simulink model "major_project1"  (R2025a)
settings: Solver=VariableStepAuto  StartTime=0.0  StopTime=5  RelTol=1e-3
undefined symbols (not defined in the file): Ion, Lithium
libraries: spsSeriesRLCBranchLib x8, spsMosfetLib x7, spsBatteryLib x3, spsVoltageMeasurementLib x3, spsPVArrayLib x1, slpidlib x1, simulink x1, spspowerguiLib x1
settings Model: Creator=Telan  LastModifiedBy=Telan
settings DataIOCC: SaveFormat=Array
settings DebuggingCC: UnderSpecifiedDimensionMsg=warning

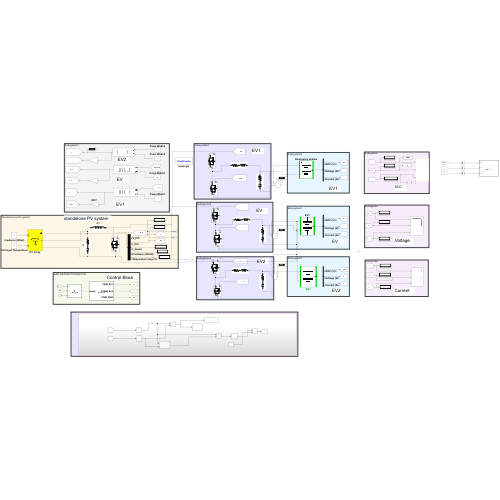
[thumbnail: Simulink's stored preview of the top-level diagram]
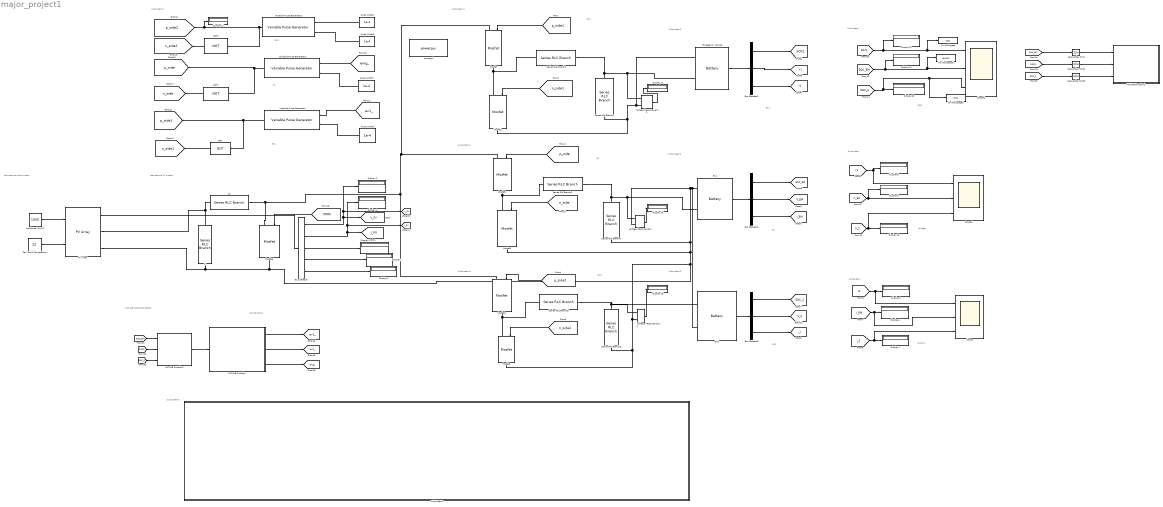
== system major_project1 ==
  note: Subsystem3
  note: EV1
  note: Subsystem
  note: Subsystem
  note: Subsystem
  note: Subsystem1
  note: MATLAB FUNCTION BLOCK
  note: Subsystem5
  note: Subsystem3
  note: Subsystem2
  note: Subsystem4
  note: Standalone solar system
  note: Subsystem4
  note: Subsystem4
  note: EV2
  note: EV
  note: EV1
  note: EV
  note: EV2
  note: SOC
  note: Voltage
  note: Current
  note: EV1
  note: EV
  note: EV2
  note: standalone PV system
  note: Control Block
  Bus Selector : BusSelector  OutputSignals=V_PV,I_PV,I_diode,Irradiance (W/m2),Temperature (deg C)
  Bus Selector1 : BusSelector  OutputSignals=SOC (%),Voltage (V),Current (A)
  Bus Selector2 : BusSelector  OutputSignals=SOC (%),Voltage (V),Current (A)
  Bus Selector3 : BusSelector  OutputSignals=SOC (%),Voltage (V),Current (A)
  C : spsSeriesRLCBranchLib/Series RLC Branch  LConnTagsString=__new0  RConnTagsString=__new0  BranchType=RC  Resistance=0.0001  Inductance=1e-3  SetiL0=off  InitialCurrent=0  Capacitance=988E-6  Setx0=off  InitialVoltage=0  Measurements=Branch voltage and current
  C1 : spsSeriesRLCBranchLib/Series RLC Branch  LConnTagsString=__new0  RConnTagsString=__new0  BranchType=L  Resistance=0.0001  Inductance=1.6e-3  SetiL0=off  InitialCurrent=0  Capacitance=988E-6  Setx0=off  InitialVoltage=0  Measurements=Branch voltage and current
  Cell Input Temperature : Constant  Value=25
  Display{,1..17} (18 alike) : Display
  EV1 : spsBatteryLib/Battery  BatType=Lithium-Ion  NomV=250  NomQ=60  SOC=30  Batt_Tr=5  PresetModel=on  MaxQ=60  MinV=187.5  FullV=290.9968  Dis_rate=26.087  R=0.041667  Normal_OP=54.2609  expZone="[270.0965      2.947826]"
  EV2 : spsBatteryLib/Battery  BatType=Lithium-Ion  NomV=250  NomQ=50  SOC=50  Batt_Tr=5  PresetModel=on  MaxQ=50  MinV=187.5  FullV=290.9968  Dis_rate=21.7391  R=0.05  Normal_OP=45.2174  expZone="[270.0965      2.456522]"
  Emergency Vehicle : spsBatteryLib/Battery  BatType=Lithium-Ion  NomV=250  NomQ=50  SOC=50  Batt_Tr=5  PresetModel=on  MaxQ=50  MinV=187.5  FullV=290.9968  Dis_rate=21.7391  R=0.05  Normal_OP=45.2174  expZone="[270.0965      2.456522]"
  Irradiance (W/m2) : Constant  Value=1000
  MATLAB Function : MATLAB Function  TreatAsAtomicUnit=on
  MATLAB Function1 : MATLAB Function  TreatAsAtomicUnit=on
  MATLAB Function2 : MATLAB Function  TreatAsAtomicUnit=on
  Mosfet{,1..6} (7 alike) : spsMosfetLib/Mosfet  Ron=0.1  Lon=0  Rd=0.01  Vfd=0  IC=0  Rs=1e5  Cs=inf  Measurements=off
  NOT : Logic  Operator=NOT  IconShape=distinctive  AllPortsSameDT=off  OutDataTypeStr=boolean
  NOT1 : Logic  Operator=NOT  IconShape=distinctive  AllPortsSameDT=off  OutDataTypeStr=boolean
  NOT2 : Logic  Operator=NOT  IconShape=distinctive  AllPortsSameDT=off  OutDataTypeStr=boolean
  PV  Array : spsPVArrayLib/PV Array  Npar=40  Nser=10  PlotType=array @ 1000 W/m2 & specified temperatures  S_vec="[ 1000  500  100 ]"  Temp_C_vec="[ 45 25  ]"  ModuleName=User-defined  PlotWhenSelected=off  Pm=213.15  Ncell=60  Voc=36.3  Isc=7.84  Vm=29  Im=7.35  beta_Voc_pc=-0.36099  alpha_Isc_pc=0.102  beta_Voc=-0.13104  alpha_Isc=0.0079968  IL=7.8654  I0=2.9273e-10  nI=0.98119  Rsh=313.0553  Rs=0.39381  RobustModel=off  RobustCellTemperature=313.3991  BAL=on  Tc=1e-6  Tfilter=5e-5
  Pulse Width{1..4} (4 alike) : Constant  Value=1e-4
  Scope : Scope  NumInputPorts=3
      settings: ActiveDisplayYMinimum=-6.4724154503791311  ActiveDisplayYMaximum=55.444981382819826
  Scope1 : Scope  NumInputPorts=3
      settings: ActiveDisplayYMinimum=-33.657064546931281  ActiveDisplayYMaximum=302.91358092238158
  Scope2 : Scope  NumInputPorts=3
      settings: ActiveDisplayYMinimum=51.5865917372177  ActiveDisplayYMaximum=51.68343264048265  DataLoggingVariableName=ScopeData2
  Series RLC Branch1 : spsSeriesRLCBranchLib/Series RLC Branch  LConnTagsString=__new0  RConnTagsString=__new0  BranchType=RL  Resistance=0.1  Inductance=9e-4  SetiL0=off  InitialCurrent=0  Capacitance=1e-6  Setx0=off  InitialVoltage=0  Measurements=None
  Series RLC Branch2 : spsSeriesRLCBranchLib/Series RLC Branch  LConnTagsString=__new0  RConnTagsString=__new0  BranchType=RC  Resistance=30  Inductance=1e-3  SetiL0=off  InitialCurrent=0  Capacitance=1e-4  Setx0=off  InitialVoltage=0  Measurements=Branch voltage
  Series RLC Branch3 : spsSeriesRLCBranchLib/Series RLC Branch  LConnTagsString=__new0  RConnTagsString=__new0  BranchType=RL  Resistance=0.1  Inductance=9e-4  SetiL0=off  InitialCurrent=0  Capacitance=1e-6  Setx0=off  InitialVoltage=0  Measurements=None
  Series RLC Branch4 : spsSeriesRLCBranchLib/Series RLC Branch  LConnTagsString=__new0  RConnTagsString=__new0  BranchType=RC  Resistance=30  Inductance=1e-3  SetiL0=off  InitialCurrent=0  Capacitance=1e-4  Setx0=off  InitialVoltage=0  Measurements=Branch voltage
  Series RLC Branch5 : spsSeriesRLCBranchLib/Series RLC Branch  LConnTagsString=__new0  RConnTagsString=__new0  BranchType=RL  Resistance=0.1  Inductance=9e-4  SetiL0=off  InitialCurrent=0  Capacitance=1e-6  Setx0=off  InitialVoltage=0  Measurements=None
  Series RLC Branch6 : spsSeriesRLCBranchLib/Series RLC Branch  LConnTagsString=__new0  RConnTagsString=__new0  BranchType=RC  Resistance=30  Inductance=1e-3  SetiL0=off  InitialCurrent=0  Capacitance=1e-4  Setx0=off  InitialVoltage=0  Measurements=Branch voltage
  Subsystem2 : Subsystem
  To Workspace : ToWorkspace  VariableName=soc1  SampleTime=1
      settings: Save2DSignal=2-D array (concatenate along first dimension)
  To Workspace1 : ToWorkspace  VariableName=soc_em  SampleTime=-1
      settings: Save2DSignal=2-D array (concatenate along first dimension)
  To Workspace2 : ToWorkspace  VariableName=soc2  SampleTime=-1
      settings: Save2DSignal=2-D array (concatenate along first dimension)
  Variable Pulse Generator : VariablePulseGenerator  AllowZeroPulseWidth=on  SampleTime=0.1
  Variable Pulse Generator1 : VariablePulseGenerator  AllowZeroPulseWidth=on  SampleTime=0.1
  Variable Pulse Generator2 : VariablePulseGenerator  AllowZeroPulseWidth=on  SampleTime=0.1
  Voltage Measurement : spsVoltageMeasurementLib/Voltage Measurement  PhasorSimulation=off  OutputType=Complex  PSBequivalent=0
  Voltage Measurement1 : spsVoltageMeasurementLib/Voltage Measurement  PhasorSimulation=off  OutputType=Complex  PSBequivalent=0
  Voltage Measurement2 : spsVoltageMeasurementLib/Voltage Measurement  PhasorSimulation=off  OutputType=Complex  PSBequivalent=0
  Zero-Order Hold : ZeroOrderHold
  Zero-Order Hold1 : ZeroOrderHold
  Zero-Order Hold2 : ZeroOrderHold
  powergui : spspowerguiLib/powergui  Priority=1  SimulationMode=Continuous  SampleTime=50e-6  frequency=60  Iterations=50  frequencyindice=0  Pbase=100e6  ErrMax=1e-4  UnitsV=kV  UnitsW=MW  buscounter=0  FunctionMessages=off  echomessages=off  EnableUseOfTLC=off  CurrentSourceSwitches=off  DisableSnubberDevices=off  DisableRonSwitches=off  DisableVfSwitches=off  DisplayEquations=off  AutomaticDiscreteSolvers=off  SolverType=Tustin/Backward Euler (TBE)  Interpol=off  ExternalGateDelay=off  methode=off  Ts=100  x0status=blocks  SPID=on  SwTol=0  HookPort=off  NonlinearTolerance=1e-4  nMaxIteration=100  ContinueOnMaxIteration=off  RestoreLinks=warning  ResistiveCurrentMeasurement=off  Frange=[0:2:500]  Ylog=off  Xlog=on  ShowGrid=off  save=off  variable=ZData  structure=0  ZoomFFT=off  StartTime=0.0  cycles=1  DisplayStyle=1  fundamental=60  FreqAxis=off  MaxFrequency=1000  frequencyindicesteady=1  RmsSteady=1  display=off
  tag scope: I1=global, I_2=global, I_EM=global, I_PV=global, SOC1=global, SOC_2=global, SOC_EM=global, V1=global, V_2=global, V_EM=global, V_PV=global, emg_=global, ev1_=global, ev2_=global, i_PV=global, n_side1=global, n_side2=global, n_side=global, p_side1=global, p_side2=global, p_side=global, v_PV=global
  wires:
  ? -> ?
  Bus Selector/3 -> Display1/1  "<I_diode>"
  Bus Selector/4 -> Display/1  "<Irradiance (W/m2)>"
  Bus Selector/5 -> Display2/1  "<Temperature (deg C)>"
  Bus Selector/2 -> [i_PV], Display4/1, [I_PV]  "<I_PV>"
  Bus Selector/1 -> Display3/1, [v_PV], [V_PV]  "<V_PV>"
  Irradiance (W/m2)/1 -> PV  Array/1
  PV  Array/1 -> Bus Selector/1
  Cell Input Temperature/1 -> PV  Array/2
  [p_side1] -> Mosfet/1
  [n_side1] -> Mosfet1/1
  [n_side] -> Mosfet3/1
  [p_side] -> Mosfet2/1
  [n_side2] -> Mosfet5/1
  [p_side2] -> Mosfet4/1
  Bus Selector1/1 -> [SOC1]  "<SOC (%)>"
  Bus Selector1/3 -> [I1]  "<Current (A)>"
  Bus Selector1/2 -> [V1]  "<Voltage (V)>"
  Emergency Vehicle/1 -> Bus Selector1/1
  Bus Selector2/1 -> [SOC_EM]  "<SOC (%)>"
  Bus Selector2/3 -> [I_EM]  "<Current (A)>"
  Bus Selector2/2 -> [V_EM]  "<Voltage (V)>"
  EV1/1 -> Bus Selector2/1
  EV2/1 -> Bus Selector3/1
  Bus Selector3/1 -> [SOC_2]  "<SOC (%)>"
  Bus Selector3/2 -> [V_2]  "<Voltage (V)>"
  Bus Selector3/3 -> [I_2]  "<Current (A)>"
  Pulse Width2/1 -> Variable Pulse Generator1/2
  NOT1/1 -> [n_side]
  Variable Pulse Generator1/1 -> NOT1/1, [p_side]
  Variable Pulse Generator/1 -> NOT/1, [p_side1]
  Pulse Width1/1 -> Variable Pulse Generator/2
  NOT2/1 -> [n_side2]
  Pulse Width3/1 -> Variable Pulse Generator2/2
  Variable Pulse Generator2/1 -> NOT2/1, Display17/1, [p_side2]
  NOT/1 -> [n_side1]
  [SOC_2] -> Display13/1, To Workspace2/1, Scope2/3
  [SOC1] -> Scope2/1, To Workspace/1, Display11/1
  [SOC_EM] -> Display12/1, To Workspace1/1, Scope2/2
  [V1] -> Scope1/1, Display8/1
  [V_2] -> Scope1/3, Display10/1
  [V_EM] -> Display9/1, Scope1/2
  [I_EM] -> Display6/1, Scope/2
  [I1] -> Display5/1, Scope/1
  [I_2] -> Scope/3, Display7/1
  MATLAB Function/1(PWM_EV1) -> [ev1_]
  MATLAB Function/2(PWM_EV2) -> [ev2_]
  MATLAB Function/3(PWM_EMG) -> [emg_]
  Voltage Measurement1/1 -> Display14/1
  Voltage Measurement/1 -> Display15/1
  Voltage Measurement2/1 -> Display16/1
  Pulse Width4/1 -> Variable Pulse Generator2/1
  [emg_] -> Variable Pulse Generator1/1
  [ev1_] -> Variable Pulse Generator/1
  [PWM] -> Mosfet6/1
  [SOC_EM] -> Zero-Order Hold/1
  [SOC1] -> Zero-Order Hold1/1
  [SOC_2] -> Zero-Order Hold2/1
  Zero-Order Hold/1 -> MATLAB Function1/1(soc_em)
  Zero-Order Hold1/1 -> MATLAB Function1/2(soc_ev1)
  Zero-Order Hold2/1 -> MATLAB Function1/3(soc_ev2)
  [SOC_EM] -> MATLAB Function2/1(soc_em)
  [SOC1] -> MATLAB Function2/2(soc_ev1)
  [SOC_2] -> MATLAB Function2/3(soc_ev2)
  MATLAB Function2/1(mode) -> MATLAB Function/1(mode)
  connections:
  Mosfet/RConn1 -- Series RLC Branch1/LConn1 -- Mosfet1/LConn1
  Series RLC Branch1/RConn1 -- Voltage Measurement1/LConn1 -- Emergency Vehicle/LConn1 -- Series RLC Branch2/LConn1
  Mosfet2/RConn1 -- Series RLC Branch3/LConn1 -- Mosfet3/LConn1
  Series RLC Branch3/RConn1 -- Voltage Measurement/LConn1 -- EV1/LConn1 -- Series RLC Branch4/LConn1
  Mosfet4/RConn1 -- Series RLC Branch5/LConn1 -- Mosfet5/LConn1
  Series RLC Branch6/LConn1 -- Series RLC Branch5/RConn1 -- EV2/LConn1 -- Voltage Measurement2/LConn1
  PV  Array/RConn1 -- C1/RConn1 -- C/LConn1
  Mosfet3/RConn1 -- C/RConn1 -- PV  Array/RConn2 -- Mosfet6/RConn1 -- Mosfet5/RConn1 -- Series RLC Branch6/RConn1 -- Voltage Measurement2/LConn2 -- EV1/LConn2 -- EV2/LConn2 -- Voltage Measurement/LConn2 -- Series RLC Branch4/RConn1
  Mosfet1/RConn1 -- Voltage Measurement1/LConn2 -- Emergency Vehicle/LConn2 -- Series RLC Branch2/RConn1
  Mosfet4/LConn1 -- Mosfet6/LConn1 -- C1/LConn1 -- Mosfet2/LConn1 -- Mosfet/LConn1

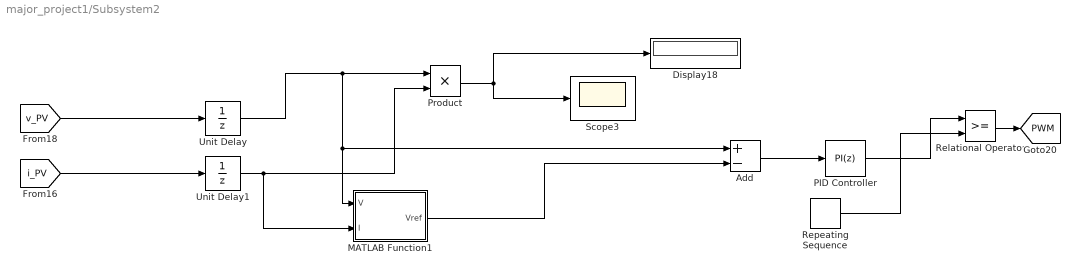
== system major_project1/Subsystem2 ==
  Add : Sum  Inputs=+-
  Display18 : Display
  MATLAB Function1 : MATLAB Function  TreatAsAtomicUnit=on
  PID Controller : slpidlib/PID Controller  Controller=PI  Form=Parallel  TimeDomain=Discrete-time  UseExternalTs=off  SampleTime=-1  IntegratorMethod=Forward Euler  FilterMethod=Forward Euler  ControllerParametersSource=internal  P=0.7  I=10  UseKiTs=off  D=0  UseExternalDerivativeSource=off  N=100  UseFilter=on  TunerSelectOption=Transfer Function Based (PID Tuner App)  InitialConditionSource=internal  InitialConditionForIntegrator=0.54  InitialConditionForFilter=0  DifferentiatorICPrevScaledInput=0  ExternalReset=none  TrackingMode=off  Kt=1  LimitOutput=on  SatLimitsSource=internal  UpperSaturationLimit=0.99  LowerSaturationLimit=0  LinearizeAsGain=on  AntiWindupMode=none  Kb=1  LimitIntegrator=off  UpperIntegratorSaturationLimit=inf  LowerIntegratorSaturationLimit=-inf  POutMin=[]  POutMax=[]  IOutMin=[]  IOutMax=[]  DOutMin=[]  DOutMax=[]  NOutMin=[]  NOutMax=[]  SumOutMin=[]  SumOutMax=[]  SaturationOutMin=[]  SaturationOutMax=[]  PParamMin=[]  PParamMax=[]  IParamMin=[]  IParamMax=[]  DParamMin=[]  DParamMax=[]  NParamMin=[]  NParamMax=[]  KbParamMin=[]  KbParamMax=[]  KtParamMin=[]  KtParamMax=[]  KbOutMin=[]  KbOutMax=[]  KtOutMin=[]  KtOutMax=[]  IntegratorOutMin=[]  IntegratorOutMax=[]  FilterOutMin=[]  FilterOutMax=[]  SumI1OutMin=[]  SumI1OutMax=[]  SumI2OutMin=[]  SumI2OutMax=[]  SumI3OutMin=[]  SumI3OutMax=[]  SumI4OutMin=[]  SumI4OutMax=[]  SumDOutMin=[]  SumDOutMax=[]  DifferentiatorOutMin=[]  DifferentiatorOutMax=[]  FilterDiffOutCoefMin=[]  FilterDiffOutCoefMax=[]  ReciprocalOutMin=[]  ReciprocalOutMax=[]  SumDenOutMin=[]  SumDenOutMax=[]  SumNumOutMin=[]  SumNumOutMax=[]  DivideOutMin=[]  DivideOutMax=[]  UdiffTsProdOutMin=[]  UdiffTsProdOutMax=[]  NTsProdOutMin=[]  NTsProdOutMax=[]  UintegralTsProdOutMin=[]  UintegralTsProdOutMax=[]  UngainTsProdOutMin=[]  UngainTsProdOutMax=[]  ClampingZeroOutDataTypeStr=Inherit: Inherit via back propagation  ClampingZeroOutMin=[]  ClampingZeroOutMax=[]  FilterDenConstantOutDataTypeStr=Inherit: Inherit via back propagation  FilterDenConstantOutMin=[]  FilterDenConstantOutMax=[]  PCopyOutDataTypeStr=Inherit: Inherit via back propagation  PCopyOutMin=[]  PCopyOutMax=[]  NCopyOutDataTypeStr=Inherit: Inherit via back propagation  NCopyOutMin=[]  NCopyOutMax=[]  IntegratorContinuousStateAttributes=''  IntegratorStateMustResolveToSignalObject=off  IntegratorRTWStateStorageClass=Auto  FilterContinuousStateAttributes=''  FilterStateMustResolveToSignalObject=off  FilterRTWStateStorageClass=Auto  ParallelPVariant=InternalParameters  IdealPVariant=Disabled  IVariant=InternalParameters  DVariant=Disabled  IntegratorVariant=Discrete  SatVariant=Enabled  AWVariant=Passthrough  PCopyVariant=Disabled  TRVariant=Disabled  FdbkBlocksVariant=Forward  IdealPFdbkVariant=Disabled  SatFdbkVariant=Disabled  DerivativeFilterVariant=Disabled  NVariant=Disabled  NCopyVariant=Disabled_SignalSpec  FilterICVariant=Disabled  IntegratorICVariant=InternalICs  ExternalResetVariant=Disabled  TRSumVariant=Passthrough  SumFdbkVariant=Disabled  SumVariant=Sum_PI  TsampFilterVariant=InternalTs  TsampNgainVariant=Passthrough  TsampIntegralVariant=Disabled_SignalSpec  ExternalSaturationOutDataTypeStr=Inherit: Same as second input  DerivativeSourceVariant=Disabled  PreIntVariant=InternalPreInt
  Product : Product
  Relational Operator : RelationalOperator  OutDataTypeStr=boolean  RndMeth=Simplest  InputSameDT=off
  Repeating Sequence : simulink/Sources/Repeating Sequence  rep_seq_t=[0 2]  rep_seq_y=[0 2]
  Scope3 : Scope
      settings: DataLoggingVariableName=ScopeData3
  Unit Delay : UnitDelay  SampleTime=-1  HasFrameUpgradeWarning=on
  Unit Delay1 : UnitDelay  SampleTime=-1  HasFrameUpgradeWarning=on
  tag scope: PWM=global
  wires:
  Relational Operator/1 -> [PWM]
  Unit Delay/1 -> Product/1, Add/1, MATLAB Function1/1(V)
  Product/1 -> Display18/1, Scope3/1
  PID Controller/1 -> Relational Operator/1
  Unit Delay1/1 -> Product/2, MATLAB Function1/2(I)
  MATLAB Function1/1(Vref) -> Add/2
  Add/1 -> PID Controller/1
  Repeating Sequence/1 -> Relational Operator/2
  [v_PV] -> Unit Delay/1
  [i_PV] -> Unit Delay1/1

== matlab function major_project1/MATLAB Function ==
  data: mode input; PWM_EV1 output; PWM_EV2 output; PWM_EMG output
function [PWM_EV1, PWM_EV2, PWM_EMG] = control_function(mode)
% mode: 1 - Normal charging
%       2 - Slower charging for EV1/EV2, fast for EMG
%       3 - Reverse charging from EV1/EV2 to EMG

% Duty cycle values (use values between 0 and 1 for Variable Pulse Generator)
PWM_fast   = 0.95;  % Fast charging (e.g., 95% duty for EMG)
PWM_normal = 0.9;  % Normal charging
PWM_slower = 0.85;  % Slower charging for EV1/EV2
PWM_reverse = 0.80; % For reverse charging

% Default assignments
PWM_EV1 = PWM_normal;
PWM_EV2 = PWM_normal;
PWM_EMG = PWM_normal;

switch mode
    case 1  % Normal charging for all
        PWM_EV1 = PWM_normal;
        PWM_EV2 = PWM_normal;
        PWM_EMG = PWM_normal;

    case 2  % Slower charging for EV1/EV2, fast for EMG
        PWM_EV1 = PWM_slower;
        PWM_EV2 = PWM_slower;
        PWM_EMG = PWM_fast;

    case 3  % Reverse charging: EV1/EV2 provide energy to EMG
        PWM_EV1 = PWM_reverse;
        PWM_EV2 = PWM_reverse;
        PWM_EMG = PWM_normal; % You may adjust this as per your setup

end
end

== matlab function major_project1/Subsystem2/MATLAB Function1 ==
  data: V input; Vref output; I input
function Vref = MPPT(V, I)

% Limits for reference voltage
Vrefmax  = 450;   % maximum PV voltage
Vrefmin  = 0;     % minimum PV voltage
Vrefinit = 400;   % initial reference
deltaVref = 1;    % step size

% Persistent variables
persistent Volt Pold Vrefold
if isempty(Volt)
    Volt = 0;
    Pold = 0;
    Vrefold = Vrefinit;
end

% Current power
P = V * I;

% Differences
dV = V - Volt;
dP = P - Pold;

% P&O algorithm
if dP ~= 0
    if dP < 0
        if dV < 0
            Vref = Vrefold + deltaVref;
        else
            Vref = Vrefold - deltaVref;
        end
    else
        if dV < 0
            Vref = Vrefold - deltaVref;
        else
            Vref = Vrefold + deltaVref;
        end
    end
else
    Vref = Vrefold;
end

% Clamp Vref between [Vrefmin, Vrefmax]
if Vref > Vrefmax
    Vref = Vrefmax;
elseif Vref < Vrefmin
    Vref = Vrefmin;
end

% Update persistent values
Volt    = V;
Pold    = P;
Vrefold = Vref;

end

== matlab function major_project1/MATLAB Function1 ==
  data: soc_em input; soc_ev1 input; soc_ev2 input
function json_export(soc_em, soc_ev1, soc_ev2)

% Tell Simulink this function runs in MATLAB, not codegen
coder.extrinsic('export_soc');

export_soc(soc_em, soc_ev1, soc_ev2);

end

== matlab function major_project1/MATLAB Function2 ==
  data: soc_em input; mode output; soc_ev1 input; soc_ev2 input
function mode = ml_mode_selector(soc_em, soc_ev1, soc_ev2)

% --- IMPORTANT: initialize output with known type ---
mode = 1;   % double scalar, default Normal mode

coder.extrinsic('py.predict_mode.predict_mode');

% Call Python only for value update
py_mode = py.predict_mode.predict_mode(soc_em, soc_ev1, soc_ev2);

% Convert Python int → MATLAB double
mode = double(py_mode);

end
